simulink model "Senorless"  (R2023a)
settings: Solver=FixedStepDiscrete  StartTime=0.0  StopTime=5  FixedStep=1/FOC_FRQ  RelTol=1e-3
values from neighbouring files (symbols this model uses):
  ADC_REF = 3.6    [Senorless.sldd]
  ADC_SAMPLE_MAX = 32767.0    [Senorless.sldd]
  AMP_GAIN = 16.0    [Senorless.sldd]
  CURR_INPUT = 3276.0    [Senorless.sldd]
  CURR_KI = 380.0    [Senorless.sldd]
  CURR_KP = 0.04    [Senorless.sldd]
  CURR_LIMIT = 0.95    [Senorless.sldd]
  CURR_OVER = 6.0    [Senorless.sldd]
  CURR_POINT_GAIN = 7.0    [Senorless.sldd]
  CURR_STEP = 32760.0    [Senorless.sldd]
  CURR_UNDER = 0.03    [Senorless.sldd]
  CURR_WIDTH = 6552.0    [Senorless.sldd]
  FOC_FRQ = 25000.0    [Senorless.sldd]
  GAMMA = 32767.0    [Senorless.sldd]
  IMAX = 10.0    [Senorless.sldd]
  LPF_FRQ = 2000.0    [Senorless.sldd]
  MOTOR_DAMPER = 2.06E-7    [Senorless.sldd]
  MOTOR_FLUX = 0.00212352    [Senorless.sldd]
  MOTOR_INERTIA = 4.0E-7    [Senorless.sldd]
  MOTOR_LS = 0.000536    [Senorless.sldd]
  MOTOR_PN = 7.0    [Senorless.sldd]
  MOTOR_RS = 4.0    [Senorless.sldd]
  OPEN_IQ = 0.28    [Senorless.sldd]
  OPEN_IQ_MIN = 0.05    [Senorless.sldd]
  OPEN_IQ_SLOW = 0.1    [Senorless.sldd]
  OPEN_SPD = 1000.0    [Senorless.sldd]
  OPEN_SPD_SLOW = 180.0    [Senorless.sldd]
  OPEN_TIME = 0.5    [Senorless.sldd]
  OPEN_TIME_NFO = 0.5    [Senorless.sldd]
  PLL_LIMIT = 0.9    [Senorless.sldd]
  PLL_WIDTH = 800.0    [Senorless.sldd]
  PWM_FRQ = 96000000.0    [Senorless.sldd]
  RS_HUNT = 0.02    [Senorless.sldd]
  SMOK_FRQ = 600.0    [Senorless.sldd]
  SPD_LIMIT = 0.9    [Senorless.sldd]
  SPD_LPF_LEVEL = 0.0    [Senorless.sldd]
  SPD_MAX = 12000.0    [Senorless.sldd]
  SPD_MIN = 4000.0    [Senorless.sldd]
  SPD_REDUCE = 380.0    [Senorless.sldd]
  SPD_STEP = 6.0    [Senorless.sldd]
  SPD_WIDTH = 20.0    [Senorless.sldd]
  THETA_ERR_LIMIT = 8192.0    [Senorless.sldd]
  TS_POINT_GAIN = 10.0    [Senorless.sldd]
  UDC = 48.0    [Senorless.sldd]
  UDC_GAIN = 21.0    [Senorless.sldd]
  UDC_POINT_GAIN = 10.0    [Senorless.sldd]
undefined symbols (not defined in the file or in its folder): curr_q_ki, curr_q_kp, DiscIntNeverNeededParam, magnitude, PLL_LPF_LEVEL, Udc
libraries: simulink x20, slpidlib x5, mcbcontrolslib x2, mcbplantlib x1, autolibpmsmexterior x1, spspowerguiLib x1
(part 5 of 8)

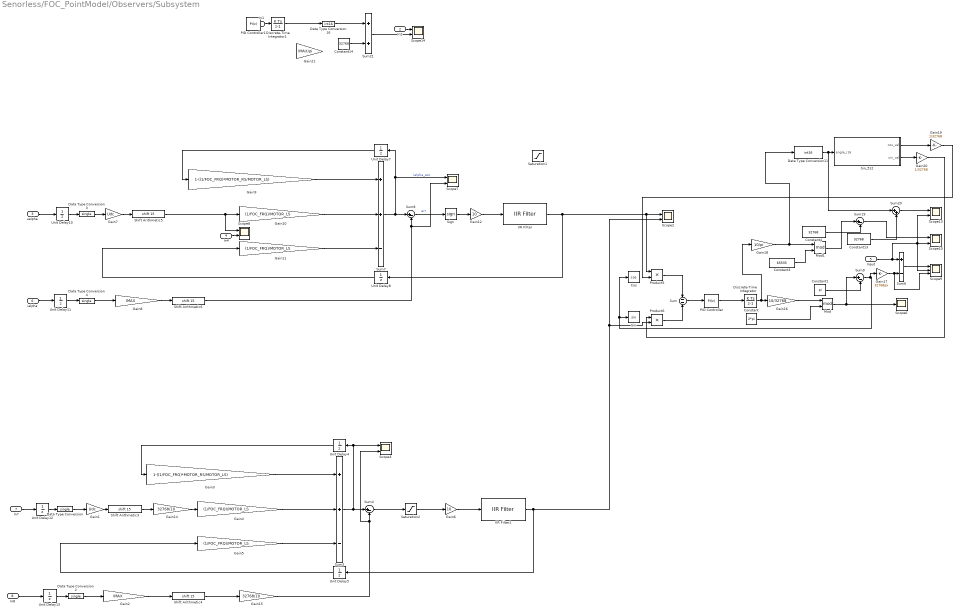
== system Senorless/FOC_PointModel/Observers/Subsystem ==
  In1 : Inport
  In2 : Inport  Port=2
  ualpha : Inport  Port=3
  In4 : Inport  Port=4
  Input : Inport  Port=5
  ialpha : Inport  Port=6
  In7 : Inport  Port=7
  In8 : Inport  Port=8
  Constant : Constant  Value=2*pi  OutDataTypeStr=single
  Constant1 : Constant  Value=pi  OutDataTypeStr=single
  Constant13 : Constant  Value=32768  OutDataTypeStr=int16
  Constant14 : Constant  Value=32768  OutDataTypeStr=int16
  Constant3 : Constant  Value=65535  OutDataTypeStr=single
  Constant4 : Constant  Value=32768
  Cos : Trigonometry  Operator=cos
  Data Type Conversion{,2..4} (4 alike) : DataTypeConversion  OutDataTypeStr=single  SaturateOnIntegerOverflow=off  RndMeth=Floor
  Data Type Conversion11 : DataTypeConversion  OutDataTypeStr=int16  SaturateOnIntegerOverflow=off  RndMeth=Floor
  Data Type Conversion16 : DataTypeConversion  OutDataTypeStr=int16  SaturateOnIntegerOverflow=off
  Discrete-Time Integrator : DiscreteIntegrator  SampleTime=-1  ICPrevOutput=DiscIntNeverNeededParam  ICPrevScaledInput=DiscIntNeverNeededParam
  Discrete-Time Integrator1 : DiscreteIntegrator  SampleTime=-1  OutDataTypeStr=int32  RndMeth=Zero  ICPrevOutput=DiscIntNeverNeededParam  ICPrevScaledInput=DiscIntNeverNeededParam
  Gain1 : Gain  Gain=Udc
  Gain10 : Gain  Gain=(1/FOC_FRQ)/MOTOR_LS
  Gain11 : Gain  Gain=(1/FOC_FRQ)/MOTOR_LS  OutDataTypeStr=single
  Gain12 : Gain  Gain=10
  Gain14 : Gain  Gain=32768/10
  Gain15 : Gain  Gain=32768/10
  Gain16 : Gain  Gain=10/32768
  Gain17 : Gain  Gain=32768/pi
  Gain18 : Gain  Gain=10/pi
  Gain19 : Gain  Gain=1/32768  OutDataTypeStr=single
  Gain2 : Gain  Gain=IMAX
  Gain20 : Gain  Gain=1/32768  OutDataTypeStr=single
  Gain21 : Gain  Gain=IMAX/pi  OutDataTypeStr=int32  RndMeth=Zero
  Gain3 : Gain  Gain=1-((1/FOC_FRQ)*MOTOR_RS/MOTOR_LS)  OutDataTypeStr=single
  Gain4 : Gain  Gain=(1/FOC_FRQ)/MOTOR_LS
  Gain5 : Gain  Gain=(1/FOC_FRQ)/MOTOR_LS  OutDataTypeStr=single
  Gain6 : Gain  Gain=10
  Gain7 : Gain  Gain=Udc
  Gain8 : Gain  Gain=IMAX
  Gain9 : Gain  Gain=1-((1/FOC_FRQ)*MOTOR_RS/MOTOR_LS)  OutDataTypeStr=single
  IIR Filter : mcbcontrolslib/IIR Filter  VariantControl=Low Pass Filter  VariantSelect=Low-pass  Filter_constant=0.1  advancedSettings=off  Ts=50e-6  cutOff_freq=353.6777
      settings: LibrarySourceBlock=mcbhdllib/Signal Management/IIR Filter
  IIR Filter1 : mcbcontrolslib/IIR Filter  VariantControl=Low Pass Filter  VariantSelect=Low-pass  Filter_constant=0.149  advancedSettings=off  Ts=50e-6  cutOff_freq=557.3228
      settings: LibrarySourceBlock=mcbhdllib/Signal Management/IIR Filter
  Mod : Math  Operator=mod
  Mod1 : Math  Operator=mod
  PID Controller : slpidlib/PID Controller  Controller=PI  Form=Parallel  TimeDomain=Discrete-time  UseExternalTs=off  SampleTime=-1  IntegratorMethod=Forward Euler  FilterMethod=Forward Euler  ControllerParametersSource=internal  P=2*0.707*100  I=100*100  UseKiTs=off  D=0  N=100  UseFilter=on  TunerSelectOption=Transfer Function Based (PID Tuner App)  InitialConditionSource=internal  InitialConditionForIntegrator=0  InitialConditionForFilter=0  DifferentiatorICPrevScaledInput=0  ExternalReset=none  TrackingMode=off  Kt=1  LimitOutput=off  SatLimitsSource=internal  UpperSaturationLimit=inf  LowerSaturationLimit=-inf  LinearizeAsGain=on  AntiWindupMode=none  Kb=1  LimitIntegrator=off  UpperIntegratorSaturationLimit=inf  LowerIntegratorSaturationLimit=-inf  POutMin=[]  POutMax=[]  IOutMin=[]  IOutMax=[]  DOutMin=[]  DOutMax=[]  NOutMin=[]  NOutMax=[]  SumOutMin=[]  SumOutMax=[]  SaturationOutMin=[]  SaturationOutMax=[]  PParamMin=[]  PParamMax=[]  IParamMin=[]  IParamMax=[]  DParamMin=[]  DParamMax=[]  NParamMin=[]  NParamMax=[]  KbParamMin=[]  KbParamMax=[]  KtParamMin=[]  KtParamMax=[]  KbOutMin=[]  KbOutMax=[]  KtOutMin=[]  KtOutMax=[]  IntegratorOutMin=[]  IntegratorOutMax=[]  FilterOutMin=[]  FilterOutMax=[]  SumI1OutMin=[]  SumI1OutMax=[]  SumI2OutMin=[]  SumI2OutMax=[]  SumI3OutMin=[]  SumI3OutMax=[]  SumI4OutMin=[]  SumI4OutMax=[]  SumDOutMin=[]  SumDOutMax=[]  DifferentiatorOutMin=[]  DifferentiatorOutMax=[]  FilterDiffOutCoefMin=[]  FilterDiffOutCoefMax=[]  ReciprocalOutMin=[]  ReciprocalOutMax=[]  SumDenOutMin=[]  SumDenOutMax=[]  SumNumOutMin=[]  SumNumOutMax=[]  DivideOutMin=[]  DivideOutMax=[]  UdiffTsProdOutMin=[]  UdiffTsProdOutMax=[]  NTsProdOutMin=[]  NTsProdOutMax=[]  UintegralTsProdOutMin=[]  UintegralTsProdOutMax=[]  UngainTsProdOutMin=[]  UngainTsProdOutMax=[]  ClampingZeroOutDataTypeStr=Inherit: Inherit via back propagation  ClampingZeroOutMin=[]  ClampingZeroOutMax=[]  FilterDenConstantOutDataTypeStr=Inherit: Inherit via back propagation  FilterDenConstantOutMin=[]  FilterDenConstantOutMax=[]  PCopyOutDataTypeStr=Inherit: Inherit via back propagation  PCopyOutMin=[]  PCopyOutMax=[]  NCopyOutDataTypeStr=Inherit: Inherit via back propagation  NCopyOutMin=[]  NCopyOutMax=[]  IntegratorContinuousStateAttributes=''  IntegratorStateMustResolveToSignalObject=off  IntegratorRTWStateStorageClass=Auto  FilterContinuousStateAttributes=''  FilterStateMustResolveToSignalObject=off  FilterRTWStateStorageClass=Auto  ParallelPVariant=InternalParameters  IdealPVariant=Disabled  IVariant=InternalParameters  DVariant=Disabled  IntegratorVariant=Discrete  SatVariant=Disabled  AWVariant=Passthrough  PCopyVariant=Disabled  TRVariant=Disabled  FdbkBlocksVariant=Forward  IdealPFdbkVariant=Disabled  SatFdbkVariant=Disabled  DerivativeFilterVariant=Disabled  NVariant=Disabled  NCopyVariant=Disabled_SignalSpec  FilterICVariant=Disabled  IntegratorICVariant=InternalICs  ExternalResetVariant=Disabled  TRSumVariant=Passthrough  SumFdbkVariant=Disabled  SumVariant=Sum_PI  TsampFilterVariant=InternalTs  TsampNgainVariant=Passthrough  TsampIntegralVariant=Disabled_SignalSpec  ExternalSaturationOutDataTypeStr=Inherit: Same as second input
  PID Controller1 : slpidlib/PID Controller  Controller=PI  Form=Parallel  TimeDomain=Discrete-time  UseExternalTs=off  SampleTime=-1  IntegratorMethod=Forward Euler  FilterMethod=Forward Euler  ControllerParametersSource=internal  P=2*0.707*100  I=100*100  UseKiTs=off  D=0  N=100  UseFilter=on  TunerSelectOption=Transfer Function Based (PID Tuner App)  InitialConditionSource=internal  InitialConditionForIntegrator=0  InitialConditionForFilter=0  DifferentiatorICPrevScaledInput=0  ExternalReset=none  TrackingMode=off  Kt=1  LimitOutput=off  SatLimitsSource=internal  UpperSaturationLimit=inf  LowerSaturationLimit=-inf  LinearizeAsGain=on  AntiWindupMode=none  Kb=1  LimitIntegrator=off  UpperIntegratorSaturationLimit=inf  LowerIntegratorSaturationLimit=-inf  PGainOutDataTypeStr=int32  PProdOutDataTypeStr=int32  POutMin=[]  POutMax=[]  IGainOutDataTypeStr=int32  IProdOutDataTypeStr=int32  IOutMin=[]  IOutMax=[]  DOutMin=[]  DOutMax=[]  NOutMin=[]  NOutMax=[]  SumOutDataTypeStr=int32  SumOutMin=[]  SumOutMax=[]  SaturationOutMin=[]  SaturationOutMax=[]  PParamDataTypeStr=int16  PParamMin=[]  PParamMax=[]  IParamDataTypeStr=int16  IParamMin=[]  IParamMax=[]  DParamMin=[]  DParamMax=[]  NParamMin=[]  NParamMax=[]  KbParamMin=[]  KbParamMax=[]  KtParamMin=[]  KtParamMax=[]  KbOutMin=[]  KbOutMax=[]  KtOutMin=[]  KtOutMax=[]  IntegratorOutDataTypeStr=int32  IntegratorOutMin=[]  IntegratorOutMax=[]  FilterOutMin=[]  FilterOutMax=[]  SumI1OutMin=[]  SumI1OutMax=[]  SumI2OutMin=[]  SumI2OutMax=[]  SumI3OutMin=[]  SumI3OutMax=[]  SumI4OutMin=[]  SumI4OutMax=[]  SumDOutMin=[]  SumDOutMax=[]  SumAccumDataTypeStr=int32  DifferentiatorOutMin=[]  DifferentiatorOutMax=[]  FilterDiffOutCoefMin=[]  FilterDiffOutCoefMax=[]  ReciprocalOutMin=[]  ReciprocalOutMax=[]  SumDenOutMin=[]  SumDenOutMax=[]  SumNumOutMin=[]  SumNumOutMax=[]  DivideOutMin=[]  DivideOutMax=[]  UdiffTsProdOutMin=[]  UdiffTsProdOutMax=[]  NTsProdOutMin=[]  NTsProdOutMax=[]  UintegralTsProdOutMin=[]  UintegralTsProdOutMax=[]  UngainTsProdOutMin=[]  UngainTsProdOutMax=[]  ClampingZeroOutDataTypeStr=Inherit: Inherit via back propagation  ClampingZeroOutMin=[]  ClampingZeroOutMax=[]  FilterDenConstantOutDataTypeStr=Inherit: Inherit via back propagation  FilterDenConstantOutMin=[]  FilterDenConstantOutMax=[]  PCopyOutDataTypeStr=Inherit: Inherit via back propagation  PCopyOutMin=[]  PCopyOutMax=[]  NCopyOutDataTypeStr=Inherit: Inherit via back propagation  NCopyOutMin=[]  NCopyOutMax=[]  IntegratorContinuousStateAttributes=''  IntegratorStateMustResolveToSignalObject=off  IntegratorRTWStateStorageClass=Auto  FilterContinuousStateAttributes=''  FilterStateMustResolveToSignalObject=off  FilterRTWStateStorageClass=Auto  ParallelPVariant=InternalParameters  IdealPVariant=Disabled  IVariant=InternalParameters  DVariant=Disabled  IntegratorVariant=Discrete  SatVariant=Disabled  AWVariant=Passthrough  PCopyVariant=Disabled  TRVariant=Disabled  FdbkBlocksVariant=Forward  IdealPFdbkVariant=Disabled  SatFdbkVariant=Disabled  DerivativeFilterVariant=Disabled  NVariant=Disabled  NCopyVariant=Disabled_SignalSpec  FilterICVariant=Disabled  IntegratorICVariant=InternalICs  ExternalResetVariant=Disabled  TRSumVariant=Passthrough  SumFdbkVariant=Disabled  SumVariant=Sum_PI  TsampFilterVariant=InternalTs  TsampNgainVariant=Passthrough  TsampIntegralVariant=Disabled_SignalSpec  ExternalSaturationOutDataTypeStr=Inherit: Same as second input
  Product5 : Product
  Product6 : Product
  Saturation1 : Saturate  UpperLimit=32768  LowerLimit=-32768
  Saturation2 : Saturate  UpperLimit=32768  LowerLimit=-32768
  Scope{2..3,7..8,10,13..14} (7 alike) : Scope  NumInputPorts=2
  Scope6 : Scope
  Scope9 : Scope  NumInputPorts=3
  Shift Arithmetic{3..6} (4 alike) : ArithShift  BitShiftNumber=15
  Sign : Signum
  Sin : Trigonometry
  Sin_512 : MATLAB Function  TreatAsAtomicUnit=on
  Sum : Sum  Inputs=--
  Sum19 : Sum  Inputs=|+-
  Sum20 : Sum  Inputs=|++
  Sum21 : Sum
  Sum3 : Sum  Inputs=++-
  Sum4 : Sum  Inputs=|+-  RndMeth=Zero
  Sum6 : Sum  Inputs=+-
  Sum7 : Sum  Inputs=++-
  Sum8 : Sum  Inputs=|+-  RndMeth=Zero
  Sum9 : Sum  Inputs=|+-
  Unit Delay{4..5,7..8,10..13} (8 alike) : UnitDelay  SampleTime=-1  HasFrameUpgradeWarning=on
  wires:
  Sum8/1 -> Sign/1  "err"
  Gain3/1 -> Sum3/1
  Sum9/1 -> Cos/1, Sin/1, Gain17/1
  Saturation2/1 -> Gain6/1
  Unit Delay11/1 -> Data Type Conversion4/1
  Sum7/1 -> Unit Delay7/1, Scope7/1, Sum8/1  "ialpha_est"
  IIR Filter1/1 -> Unit Delay5/1, Scope2/2, Product6/2
  Data Type Conversion4/1 -> Gain8/1
  Unit Delay10/1 -> Data Type Conversion3/1
  Gain18/1 -> Mod1/1, Data Type Conversion11/1
  Gain20/1 -> Product6/1
  Sin_512/1(cos_val) -> Gain19/1
  Product5/1 -> Sum/1
  Gain15/1 -> Scope3/2, Sum4/2
  Sum4/1 -> Saturation2/1
  Input/1 -> Scope13/2, Scope9/2, Scope10/2, Sum6/1
  Gain4/1 -> Sum3/2
  Shift Arithmetic3/1 -> Gain14/1
  Gain2/1 -> Shift Arithmetic4/1
  Shift Arithmetic5/1 -> Scope8/1, Gain10/1
  Sum3/1 -> Scope3/1, Unit Delay4/1, Sum4/1
  Data Type Conversion3/1 -> Gain7/1
  Constant14/1 -> Sum21/2
  Unit Delay4/1 -> Gain3/1
  Gain1/1 -> Shift Arithmetic3/1
  Gain10/1 -> Sum7/2
  Discrete-Time Integrator1/1 -> Data Type Conversion16/1
  Sum21/1 -> Scope14/2
  Shift Arithmetic6/1 -> Scope7/2, Sum8/2
  Data Type Conversion/1 -> Gain1/1
  Shift Arithmetic4/1 -> Gain15/1
  Sign/1 -> Gain12/1
  Constant3/1 -> Mod1/2
  Gain8/1 -> Shift Arithmetic6/1
  Gain11/1 -> Sum7/3
  Unit Delay12/1 -> Data Type Conversion/1
  ialpha/1 -> Unit Delay11/1
  Unit Delay7/1 -> Gain9/1
  Unit Delay13/1 -> Data Type Conversion2/1
  Data Type Conversion2/1 -> Gain2/1
  Sum19/1 -> Scope10/1
  Gain5/1 -> Sum3/3
  Gain7/1 -> Shift Arithmetic5/1
  Constant/1 -> Mod/2
  Unit Delay5/1 -> Gain5/1
  ualpha/1 -> Unit Delay10/1
  Unit Delay8/1 -> Gain11/1
  Gain9/1 -> Sum7/1
  Mod/1 -> Sum9/1, Scope6/1
  Discrete-Time Integrator/1 -> Gain18/1, Gain16/1
  Gain17/1 -> Scope9/3, Sum6/2
  Constant4/1 -> Sum19/2
  IIR Filter/1 -> Unit Delay8/1, Product5/1, Scope2/1
  PID Controller/1 -> Discrete-Time Integrator/1
  Gain16/1 -> Mod/1
  Data Type Conversion16/1 -> Sum21/1
  Sin_512/2(sin_val) -> Gain20/1
  Constant1/1 -> Sum9/2
  Mod1/1 -> Sum19/1
  Gain19/1 -> Product5/2
  Constant13/1 -> Sum20/2
  Sum6/1 -> Scope9/1
  Gain6/1 -> IIR Filter1/1
  Data Type Conversion11/1 -> Sum20/1, Sin_512/1(angle_i16)
  Gain12/1 -> IIR Filter/1
  Sum20/1 -> Scope13/1
  Gain14/1 -> Gain4/1
  In2/1 -> Scope14/1
  Product6/1 -> Sum/2
  Sum/1 -> PID Controller/1
  In4/1 -> Scope8/2
  In7/1 -> Unit Delay12/1
  In8/1 -> Unit Delay13/1
  In1/1 -> Discrete-Time Integrator1/1

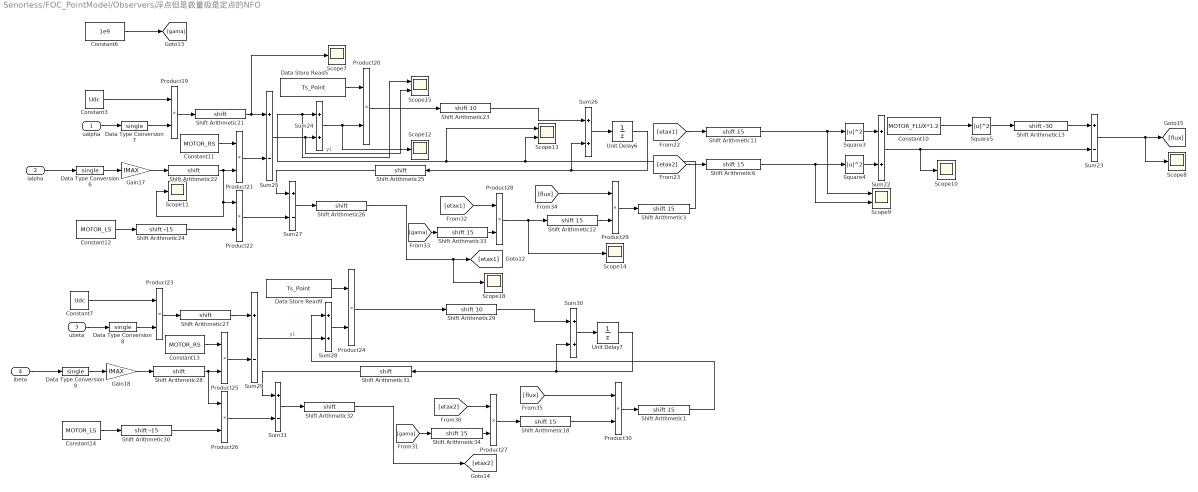
== system Senorless/FOC_PointModel/Observers/浮点但是数量级是定点的NFO ==
  ualpha : Inport
  ialpha : Inport  Port=2
  ubeta : Inport  Port=3
  ibeta : Inport  Port=4
  Constant10 : Constant  Value=MOTOR_FLUX*1.2  OutDataTypeStr=single
  Constant11 : Constant  Value=MOTOR_RS  OutDataTypeStr=single
  Constant12 : Constant  Value=MOTOR_LS  OutDataTypeStr=single
  Constant13 : Constant  Value=MOTOR_RS  OutDataTypeStr=single
  Constant14 : Constant  Value=MOTOR_LS  OutDataTypeStr=single
  Constant3 : Constant  Value=Udc  OutDataTypeStr=single
  Constant6 : Constant  Value=1e9  OutDataTypeStr=uint32
  Constant7 : Constant  Value=Udc  OutDataTypeStr=single
  Data Store Read5 : DataStoreRead  DataStoreName=Ts_Point  IndexOptions=Index vector (dialog)  Indices=1  OutputSizes=1
  Data Store Read9 : DataStoreRead  DataStoreName=Ts_Point  IndexOptions=Index vector (dialog)  Indices=1  OutputSizes=1
  Data Type Conversion{6..9} (4 alike) : DataTypeConversion  OutDataTypeStr=single  SaturateOnIntegerOverflow=off  RndMeth=Floor
  Gain17 : Gain  Gain=IMAX  ParamDataTypeStr=single  OutDataTypeStr=single  RndMeth=Zero
  Gain18 : Gain  Gain=IMAX  ParamDataTypeStr=int16  OutDataTypeStr=single  RndMeth=Zero
  Product{19..30} (12 alike) : Product  OutDataTypeStr=single  RndMeth=Zero
  Scope{7..8,10..12,14,18} (7 alike) : Scope
  Scope13 : Scope  NumInputPorts=2
  Scope15 : Scope  NumInputPorts=2
  Scope9 : Scope  NumInputPorts=2
  Shift Arithmetic{1,3,6,11..12,18,33..34} (8 alike) : ArithShift  BitShiftNumber=15
  Shift Arithmetic13 : ArithShift  BitShiftNumber=-30
  Shift Arithmetic{21..22,25..28,31..32} (8 alike) : ArithShift
  Shift Arithmetic23 : ArithShift  BitShiftNumber=10
  Shift Arithmetic24 : ArithShift  BitShiftNumber=-15
  Shift Arithmetic29 : ArithShift  BitShiftNumber=10
  Shift Arithmetic30 : ArithShift  BitShiftNumber=-15
  Square3 : Math  Operator=magnitude^2
  Square4 : Math  Operator=magnitude^2
  Square5 : Math  Operator=magnitude^2
  Sum{22,24,26,28,30} (5 alike) : Sum  OutDataTypeStr=single  RndMeth=Zero
  Sum{23,25,27,29,31} (5 alike) : Sum  Inputs=+-  OutDataTypeStr=single  RndMeth=Zero
  Unit Delay6 : UnitDelay  SampleTime=-1  HasFrameUpgradeWarning=on
  Unit Delay7 : UnitDelay  SampleTime=-1  HasFrameUpgradeWarning=on
  wires:
  Product25/1 -> Sum29/2
  Shift Arithmetic29/1 -> Sum30/1
  Product24/1 -> Shift Arithmetic29/1
  Product26/1 -> Sum31/2
  Unit Delay6/1 -> Sum26/2, Shift Arithmetic25/1
  Gain17/1 -> Shift Arithmetic22/1
  Shift Arithmetic11/1 -> Scope9/1, Square3/1
  Constant7/1 -> Product23/1
  Shift Arithmetic13/1 -> Sum23/1
  Gain18/1 -> Shift Arithmetic28/1
  Sum31/1 -> Shift Arithmetic32/1
  Shift Arithmetic3/1 -> Scope13/1, Scope15/1, Sum24/1, Scope13/2
  Shift Arithmetic28/1 -> Product26/1, Product25/2
  Unit Delay7/1 -> Sum30/2, Shift Arithmetic31/1
  Sum22/1 -> Scope10/1, Sum23/2
  Sum29/1 -> Sum28/2  "y1"
  Data Type Conversion6/1 -> Gain17/1
  Shift Arithmetic27/1 -> Sum29/1
  [flux] -> Product30/1
  Data Type Conversion8/1 -> Product23/2
  Shift Arithmetic23/1 -> Sum26/1
  Constant13/1 -> Product25/1
  Sum23/1 -> Scope8/1, [flux]
  Product27/1 -> Shift Arithmetic18/1
  Data Store Read9/1 -> Product24/1
  Sum28/1 -> Product24/2
  Sum24/1 -> Scope12/1, Product20/2
  Constant14/1 -> Shift Arithmetic30/1
  Sum30/1 -> Unit Delay7/1
  Shift Arithmetic25/1 -> Sum27/1
  Constant12/1 -> Shift Arithmetic24/1
  Shift Arithmetic31/1 -> Sum31/1
  Constant3/1 -> Product19/1
  Product23/1 -> Shift Arithmetic27/1
  Shift Arithmetic6/1 -> Scope9/2, Square4/1
  Shift Arithmetic34/1 -> Product27/2
  Square5/1 -> Shift Arithmetic13/1
  Square3/1 -> Sum22/1
  Product19/1 -> Shift Arithmetic21/1
  Sum26/1 -> Unit Delay6/1
  [etax1] -> Product28/1
  Sum27/1 -> Shift Arithmetic26/1
  Product29/1 -> Shift Arithmetic3/1
  Shift Arithmetic12/1 -> Product29/2
  ibeta/1 -> Data Type Conversion9/1
  [flux] -> Product29/1
  Constant11/1 -> Product21/1
  Product28/1 -> Scope14/1, Shift Arithmetic12/1
  Product22/1 -> Sum27/2
  Shift Arithmetic32/1 -> [etax2]
  Product21/1 -> Sum25/2
  Shift Arithmetic22/1 -> Product22/1, Scope11/1, Product21/2
  Shift Arithmetic33/1 -> Product28/2
  Sum25/1 -> Scope15/2, Sum24/2  "y1"
  [gama] -> Shift Arithmetic34/1
  Square4/1 -> Sum22/2
  Product20/1 -> Shift Arithmetic23/1
  ualpha/1 -> Data Type Conversion7/1
  [gama] -> Shift Arithmetic33/1
  Constant10/1 -> Square5/1
  Shift Arithmetic18/1 -> Product30/2
  Shift Arithmetic26/1 -> Scope18/1, [etax1]
  [etax2] -> Product27/1
  [etax1] -> Shift Arithmetic11/1
  Data Type Conversion9/1 -> Gain18/1
  ialpha/1 -> Data Type Conversion6/1
  Shift Arithmetic21/1 -> Scope7/1, Sum25/1
  Shift Arithmetic30/1 -> Product26/2
  Product30/1 -> Shift Arithmetic1/1
  Shift Arithmetic24/1 -> Product22/2
  [etax2] -> Shift Arithmetic6/1
  Shift Arithmetic1/1 -> Sum28/1
  Data Type Conversion7/1 -> Product19/2
  ubeta/1 -> Data Type Conversion8/1
  Data Store Read5/1 -> Product20/1
  Constant6/1 -> [gama]

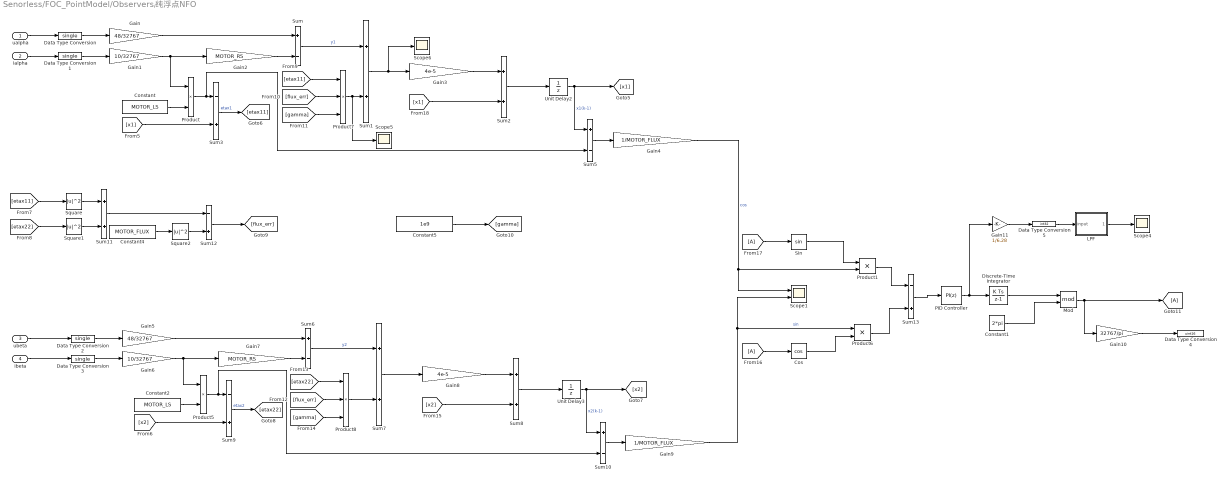
== system Senorless/FOC_PointModel/Observers/纯浮点NFO ==
  ualpha : Inport
  ialpha : Inport  Port=2
  ubeta : Inport  Port=3
  ibeta : Inport  Port=4
  Constant : Constant  Value=MOTOR_LS
  Constant1 : Constant  Value=2*pi  OutDataTypeStr=single
  Constant2 : Constant  Value=MOTOR_LS
  Constant4 : Constant  Value=MOTOR_FLUX
  Constant5 : Constant  Value=1e9  OutDataTypeStr=single
  Cos : Trigonometry  Operator=cos
  Data Type Conversion{,1..3} (4 alike) : DataTypeConversion  OutDataTypeStr=single  SaturateOnIntegerOverflow=off  RndMeth=Floor
  Data Type Conversion4 : DataTypeConversion  OutDataTypeStr=uint16  SaturateOnIntegerOverflow=off  RndMeth=Floor
  Data Type Conversion5 : DataTypeConversion  OutDataTypeStr=int32  SaturateOnIntegerOverflow=off  RndMeth=Floor
  Discrete-Time Integrator : DiscreteIntegrator  SampleTime=-1  ICPrevOutput=DiscIntNeverNeededParam  ICPrevScaledInput=DiscIntNeverNeededParam
  From16 : From
  From17 : From
  Gain : Gain  Gain=48/32767
  Gain1 : Gain  Gain=10/32767
  Gain10 : Gain  Gain=32767/pi
  Gain11 : Gain  Gain=1/6.28
  Gain2 : Gain  Gain=MOTOR_RS
  Gain3 : Gain  Gain=4e-5  OutDataTypeStr=single
  Gain4 : Gain  Gain=1/MOTOR_FLUX
  Gain5 : Gain  Gain=48/32767
  Gain6 : Gain  Gain=10/32767
  Gain7 : Gain  Gain=MOTOR_RS
  Gain8 : Gain  Gain=4e-5  OutDataTypeStr=single
  Gain9 : Gain  Gain=1/MOTOR_FLUX
  Goto11 : Goto
  LPF : Subsystem  TreatAsAtomicUnit=on
  Mod : Math  Operator=mod
  PID Controller : slpidlib/PID Controller  Controller=PI  Form=Parallel  TimeDomain=Discrete-time  UseExternalTs=off  SampleTime=-1  IntegratorMethod=Forward Euler  FilterMethod=Forward Euler  ControllerParametersSource=internal  P=2*800  I=800*800  UseKiTs=off  D=0  N=100  UseFilter=on  TunerSelectOption=Transfer Function Based (PID Tuner App)  InitialConditionSource=internal  InitialConditionForIntegrator=0  InitialConditionForFilter=0  DifferentiatorICPrevScaledInput=0  ExternalReset=none  TrackingMode=off  Kt=1  LimitOutput=off  SatLimitsSource=internal  UpperSaturationLimit=inf  LowerSaturationLimit=-inf  LinearizeAsGain=on  AntiWindupMode=none  Kb=1  LimitIntegrator=off  UpperIntegratorSaturationLimit=inf  LowerIntegratorSaturationLimit=-inf  POutMin=[]  POutMax=[]  IOutMin=[]  IOutMax=[]  DOutMin=[]  DOutMax=[]  NOutMin=[]  NOutMax=[]  SumOutMin=[]  SumOutMax=[]  SaturationOutMin=[]  SaturationOutMax=[]  PParamMin=[]  PParamMax=[]  IParamMin=[]  IParamMax=[]  DParamMin=[]  DParamMax=[]  NParamMin=[]  NParamMax=[]  KbParamMin=[]  KbParamMax=[]  KtParamMin=[]  KtParamMax=[]  KbOutMin=[]  KbOutMax=[]  KtOutMin=[]  KtOutMax=[]  IntegratorOutMin=[]  IntegratorOutMax=[]  FilterOutMin=[]  FilterOutMax=[]  SumI1OutMin=[]  SumI1OutMax=[]  SumI2OutMin=[]  SumI2OutMax=[]  SumI3OutMin=[]  SumI3OutMax=[]  SumI4OutMin=[]  SumI4OutMax=[]  SumDOutMin=[]  SumDOutMax=[]  DifferentiatorOutMin=[]  DifferentiatorOutMax=[]  FilterDiffOutCoefMin=[]  FilterDiffOutCoefMax=[]  ReciprocalOutMin=[]  ReciprocalOutMax=[]  SumDenOutMin=[]  SumDenOutMax=[]  SumNumOutMin=[]  SumNumOutMax=[]  DivideOutMin=[]  DivideOutMax=[]  UdiffTsProdOutMin=[]  UdiffTsProdOutMax=[]  NTsProdOutMin=[]  NTsProdOutMax=[]  UintegralTsProdOutMin=[]  UintegralTsProdOutMax=[]  UngainTsProdOutMin=[]  UngainTsProdOutMax=[]  ClampingZeroOutDataTypeStr=Inherit: Inherit via back propagation  ClampingZeroOutMin=[]  ClampingZeroOutMax=[]  FilterDenConstantOutDataTypeStr=Inherit: Inherit via back propagation  FilterDenConstantOutMin=[]  FilterDenConstantOutMax=[]  PCopyOutDataTypeStr=Inherit: Inherit via back propagation  PCopyOutMin=[]  PCopyOutMax=[]  NCopyOutDataTypeStr=Inherit: Inherit via back propagation  NCopyOutMin=[]  NCopyOutMax=[]  IntegratorContinuousStateAttributes=''  IntegratorStateMustResolveToSignalObject=off  IntegratorRTWStateStorageClass=Auto  FilterContinuousStateAttributes=''  FilterStateMustResolveToSignalObject=off  FilterRTWStateStorageClass=Auto  ParallelPVariant=InternalParameters  IdealPVariant=Disabled  IVariant=InternalParameters  DVariant=Disabled  IntegratorVariant=Discrete  SatVariant=Disabled  AWVariant=Passthrough  PCopyVariant=Disabled  TRVariant=Disabled  FdbkBlocksVariant=Forward  IdealPFdbkVariant=Disabled  SatFdbkVariant=Disabled  DerivativeFilterVariant=Disabled  NVariant=Disabled  NCopyVariant=Disabled_SignalSpec  FilterICVariant=Disabled  IntegratorICVariant=InternalICs  ExternalResetVariant=Disabled  TRSumVariant=Passthrough  SumFdbkVariant=Disabled  SumVariant=Sum_PI  TsampFilterVariant=InternalTs  TsampNgainVariant=Passthrough  TsampIntegralVariant=Disabled_SignalSpec  ExternalSaturationOutDataTypeStr=Inherit: Same as second input
  Product{,1,5..6} (4 alike) : Product
  Product7 : Product  Inputs=3
  Product8 : Product  Inputs=3
  Scope1 : Scope  NumInputPorts=2
  Scope4 : Scope
  Scope5 : Scope
  Scope6 : Scope
  Sin : Trigonometry
  Square : Math  Operator=magnitude^2  OutputSignalType=real
  Square1 : Math  Operator=magnitude^2  OutputSignalType=real
  Square2 : Math  Operator=magnitude^2  OutputSignalType=real
  Sum{,5..6,10} (4 alike) : Sum  Inputs=+-
  Sum{1..2,7..8,11} (5 alike) : Sum
  Sum{3,9,12..13} (4 alike) : Sum  Inputs=-+
  Unit Delay2 : UnitDelay  SampleTime=-1  HasFrameUpgradeWarning=on
  Unit Delay3 : UnitDelay  SampleTime=-1  HasFrameUpgradeWarning=on
  wires:
  Gain8/1 -> Sum8/1
  Constant2/1 -> Product5/2
  Sum/1 -> Sum1/1  "y1"
  Sum2/1 -> Unit Delay2/1
  Sum10/1 -> Gain9/1
  Gain4/1 -> Scope1/1, Product1/2  "cos"
  [x1] -> Sum2/2
  ibeta/1 -> Data Type Conversion3/1
  ubeta/1 -> Data Type Conversion2/1
  [etax22] -> Square1/1
  Data Type Conversion/1 -> Gain/1
  [etax11] -> Square/1
  Sum9/1 -> [etax22]  "etax2"
  Gain/1 -> Sum/1
  Product5/1 -> Sum10/2, Sum9/1
  Square2/1 -> Sum12/2
  Product1/1 -> Sum13/1
  Gain5/1 -> Sum6/1
  Sum1/1 -> Scope6/1, Gain3/1
  Data Type Conversion3/1 -> Gain6/1
  Sum8/1 -> Unit Delay3/1
  [flux_err] -> Product8/2
  Sum5/1 -> Gain4/1
  PID Controller/1 -> Gain11/1, Discrete-Time Integrator/1
  Cos/1 -> Product6/2
  [etax22] -> Product8/1
  [gamma] -> Product7/3
  Square1/1 -> Sum11/2
  [x1] -> Sum3/2
  Constant/1 -> Product/2
  Product7/1 -> Scope5/1, Sum1/2
  Sum13/1 -> PID Controller/1
  Square/1 -> Sum11/1
  Sum6/1 -> Sum7/1  "y2"
  Product8/1 -> Sum7/2
  Discrete-Time Integrator/1 -> Mod/1
  [flux_err] -> Product7/2
  Constant5/1 -> [gamma]
  Constant4/1 -> Square2/1
  Sum12/1 -> [flux_err]
  [gamma] -> Product8/3
  Sum3/1 -> [etax11]  "etax1"
  Gain9/1 -> Scope1/2, Product6/1  "sin"
  [etax11] -> Product7/1
  Gain7/1 -> Sum6/2
  Gain1/1 -> Product/1, Gain2/1
  Gain10/1 -> Data Type Conversion4/1
  ialpha/1 -> Data Type Conversion1/1
  Gain6/1 -> Gain7/1, Product5/1
  Gain3/1 -> Sum2/1
  Sin/1 -> Product1/1
  Product6/1 -> Sum13/2
  Sum11/1 -> Sum12/1
  From17/1 -> Sin/1
  Data Type Conversion1/1 -> Gain1/1
  Gain11/1 -> Data Type Conversion5/1
  Mod/1 -> Gain10/1, Goto11/1
  From16/1 -> Cos/1
  Constant1/1 -> Mod/2
  [x2] -> Sum8/2
  Gain2/1 -> Sum/2
  [x2] -> Sum9/2
  Data Type Conversion2/1 -> Gain5/1
  Sum7/1 -> Gain8/1
  Unit Delay3/1 -> Sum10/1, [x2]  "x2(k-1)"
  Unit Delay2/1 -> Sum5/1, [x1]  "x1(k-1)"
  Product/1 -> Sum5/2, Sum3/1
  LPF/1(output) -> Scope4/1
  Data Type Conversion5/1 -> LPF/1(input)
  ualpha/1 -> Data Type Conversion/1

== system Senorless/FOC_PointModel/SVPWM/AntiClark ==
  note: Va = Valpha;
      | Vb = Valpha*(-1/2)+Vbeta*sqrt(3)/2
      | Vc = Valpha*(-1/2)-Vbeta*sqrt(3)/2
  Valpha : Inport
  Vbeta : Inport  Port=2
  Gain1 : Gain  Gain=32767*sqrt(3)/2  ParamDataTypeStr=int16  OutDataTypeStr=int32  RndMeth=Zero
  Shift Arithmetic : ArithShift  BitShiftNumber=15
  Shift Arithmetic1 : ArithShift  BitShiftNumber=1
  Sum : Sum  Inputs=|-+  RndMeth=Zero
  Sum1 : Sum  Inputs=--|  RndMeth=Zero
  Va : Outport
  Vb : Outport  Port=2
  Vc : Outport  Port=3
  wires:
  Vbeta/1 -> Gain1/1
  Shift Arithmetic1/1 -> Sum1/2, Sum/1
  Sum/1 -> Vb/1
  Gain1/1 -> Shift Arithmetic/1
  Sum1/1 -> Vc/1
  Shift Arithmetic/1 -> Sum1/1, Sum/2
  Valpha/1 -> Va/1, Shift Arithmetic1/1

== system Senorless/FOC_PointModel/SVPWM/ei_t ==
  note: V0 = -1/2(Vmax+Vmin)
  Vabc : Inport
  Demux : Demux  Outputs=3
  Min : MinMax  Inputs=3  RndMeth=Zero
  Min1 : MinMax  Function=max  Inputs=3  RndMeth=Zero
  Shift Arithmetic : ArithShift  BitShiftNumber=1
  Sum : Sum  Inputs=|++  OutDataTypeStr=int32  RndMeth=Zero
  Unary Minus : UnaryMinus
  ei_t : Outport
  wires:
  Min/1 -> Sum/1
  Sum/1 -> Shift Arithmetic/1
  Min1/1 -> Sum/2
  Shift Arithmetic/1 -> Unary Minus/1
  Vabc/1 -> Demux/1
  Demux/1 -> Min1/1, Min/1
  Demux/2 -> Min/2, Min1/2
  Demux/3 -> Min1/3, Min/3
  Unary Minus/1 -> ei_t/1

== system Senorless/FOC_PointModel/idq_Controller/PI Controller ==
  input : Inport
  Kp : Inport  Port=2
  Ki : Inport  Port=3
  Data Store Read3 : DataStoreRead  DataStoreName=Curr_Limit  IndexOptions=Index vector (dialog)  Indices=1  OutputSizes=1
  Gain : Gain  Gain=-1  OutDataTypeStr=int32  RndMeth=Zero
  Product2 : Product  OutDataTypeStr=int32  RndMeth=Zero
  Saturation Dynamic2 : simulink/Discontinuities/Saturation Dynamic  OutMin=[]  OutMax=[]  OutDataTypeStr=Inherit: Same as second input  OutDataType=fixdt(1, 16)  OutScaling=2^-10  RndMeth=Zero  DoSatur=off
  Scope : Scope  NumInputPorts=2
  Sum : Sum  OutDataTypeStr=int32  RndMeth=Zero
  input1 : InportShadow
  积分器 : Subsystem
      settings: MinAlgLoopOccurrences=on
  output : Outport
  wires:
  input/1 -> Product2/1
  Kp/1 -> Product2/2
  Ki/1 -> 积分器/1(Ki)
  input1/1 -> 积分器/2(input)
  Product2/1 -> Scope/1, Sum/1
  积分器/1(output) -> Sum/2, Scope/2
  Sum/1 -> Saturation Dynamic2/2
  Saturation Dynamic2/1 -> output/1
  Data Store Read3/1 -> [limit]
  [limit] -> Gain/1
  Gain/1 -> Saturation Dynamic2/3
  [limit] -> Saturation Dynamic2/1

== system Senorless/FOC_PointModel/idq_Controller/PI Controller1 ==
  Ki : Inport
  Kp : Inport  Port=2
  input : Inport  Port=3
  Data Store Read3 : DataStoreRead  DataStoreName=Curr_Limit  IndexOptions=Index vector (dialog)  Indices=1  OutputSizes=1
  Gain : Gain  Gain=-1  OutDataTypeStr=int32  RndMeth=Zero
  Product2 : Product  OutDataTypeStr=int32  RndMeth=Zero
  Saturation Dynamic2 : simulink/Discontinuities/Saturation Dynamic  OutMin=[]  OutMax=[]  OutDataTypeStr=Inherit: Same as second input  OutDataType=fixdt(1, 16)  OutScaling=2^-10  RndMeth=Zero  DoSatur=off
  Scope : Scope  NumInputPorts=2
  Sum : Sum  OutDataTypeStr=int32  RndMeth=Zero
  input1 : InportShadow  Port=3
  积分器 : Subsystem
      settings: MinAlgLoopOccurrences=on
  output : Outport
  wires:
  [limit] -> Saturation Dynamic2/1
  Gain/1 -> Saturation Dynamic2/3
  [limit] -> Gain/1
  Data Store Read3/1 -> [limit]
  Saturation Dynamic2/1 -> output/1
  Sum/1 -> Saturation Dynamic2/2
  积分器/1(output) -> Scope/2, Sum/2
  Product2/1 -> Sum/1, Scope/1
  input1/1 -> 积分器/2(input)
  Ki/1 -> 积分器/1(Ki)
  Kp/1 -> Product2/2
  input/1 -> Product2/1

== system Senorless/FOC_PointModel/idq_Controller/PI Controller2 ==
  input : Inport
  Kp : Inport  Port=2
  Ki : Inport  Port=3
  Reset : Inport  Port=4
  Xo : Inport  Port=5
  Action Port : ActionPort  InitializeStates=reset  ActionPortLabel=if(u1 > 0)
  Data Store Read3 : DataStoreRead  DataStoreName=Curr_Limit  IndexOptions=Index vector (dialog)  Indices=1  OutputSizes=1
  Gain : Gain  Gain=-1  OutDataTypeStr=int32  RndMeth=Zero
  MATLAB Function : MATLAB Function  TreatAsAtomicUnit=on
  Product2 : Product  OutDataTypeStr=int32  RndMeth=Zero
  Scope : Scope  NumInputPorts=2
  Sum : Sum  OutDataTypeStr=int32  RndMeth=Zero
  input1 : InportShadow
  积分器/双边沿初始化 : Subsystem
      settings: MinAlgLoopOccurrences=on
  output : Outport
  wires:
  [limit] -> MATLAB Function/2(up), Gain/1
  Gain/1 -> MATLAB Function/3(low)
  Data Store Read3/1 -> [limit]
  MATLAB Function/1(out) -> output/1
  Sum/1 -> MATLAB Function/1(in)
  积分器/双边沿初始化/1(output) -> Scope/2, Sum/2
  Product2/1 -> Sum/1, Scope/1
  input1/1 -> 积分器/双边沿初始化/2(input)
  Reset/1 -> 积分器/双边沿初始化/4(Reset)
  Xo/1 -> 积分器/双边沿初始化/3(Xo)
  Ki/1 -> 积分器/双边沿初始化/1(Ki)
  Kp/1 -> Product2/2
  input/1 -> Product2/1

== system Senorless/FOC_PointModel/加速强拖/FreqGenerator_point2 ==
  Freq : Inport
  Reset : Inport  Port=2
  Constant : Constant  Value=32768  OutDataTypeStr=int16
  Data Type Conversion : DataTypeConversion  OutDataTypeStr=int16  SaturateOnIntegerOverflow=off
  Data Type Conversion1 : DataTypeConversion  OutDataTypeStr=int16  SaturateOnIntegerOverflow=off
  Discrete-Time Integrator : DiscreteIntegrator  ExternalReset=rising  SampleTime=-1  OutDataTypeStr=int32  RndMeth=Zero  ICPrevOutput=DiscIntNeverNeededParam  ICPrevScaledInput=DiscIntNeverNeededParam
  Discrete-Time Integrator1 : DiscreteIntegrator  ExternalReset=rising  SampleTime=-1  OutDataTypeStr=int32  RndMeth=Zero  ICPrevOutput=DiscIntNeverNeededParam  ICPrevScaledInput=DiscIntNeverNeededParam
  Gain6 : Gain  Gain=65535  OutDataTypeStr=int32  RndMeth=Zero
  Scope : Scope
  Scope1 : Scope
  Scope2 : Scope
  Shift Arithmetic : ArithShift  BitShiftNumber=-8
  Shift Arithmetic1 : ArithShift  BitShiftNumber=8
  Theta : Outport
  wires:
  Freq/1 -> Data Type Conversion1/1
  Gain6/1 -> Shift Arithmetic/1
  Data Type Conversion1/1 -> Gain6/1
  Discrete-Time Integrator/1 -> Scope2/1, Scope/1, Shift Arithmetic1/1
  Shift Arithmetic1/1 -> Data Type Conversion/1
  Reset/1 -> Discrete-Time Integrator1/2, Discrete-Time Integrator/2
  Discrete-Time Integrator1/1 -> Scope1/1, Discrete-Time Integrator/1
  Shift Arithmetic/1 -> Discrete-Time Integrator1/1
  Data Type Conversion/1 -> Theta/1

== system Senorless/FOC_PointModel/加速强拖/Subsystem ==
  Open_Hz : Inport
  Reset : Inport  Port=2
  Constant1 : Constant  Value=0  OutDataTypeStr=int32
  Gain : Gain  Gain=256  OutDataTypeStr=int32  RndMeth=Zero
  Saturation : Saturate  UpperLimit=1  LowerLimit=-1
  Sum : Sum  Inputs=-+|
  Sum1 : Sum  Inputs=++|  RndMeth=Zero
  Switch : Switch  Threshold=1  OutDataTypeStr=int32  RndMeth=Zero  SaturateOnIntegerOverflow=off  InputSameDT=off
  Unit Delay : UnitDelay  SampleTime=-1  HasFrameUpgradeWarning=on
  Out1 : Outport
  wires:
  Unit Delay/1 -> Sum1/1, Sum/1
  Gain/1 -> Sum/2
  Switch/1 -> Out1/1, Unit Delay/1
  Saturation/1 -> Sum1/2
  Sum/1 -> Saturation/1
  Constant1/1 -> Switch/3
  Open_Hz/1 -> Gain/1
  Sum1/1 -> Switch/1
  Reset/1 -> Switch/2

== system Senorless/FOC_PointModel/加速强拖/加速积分角度 ==
  Acc : Inport
  Data Type Conversion : DataTypeConversion  Commented=on  OutDataTypeStr=int16  SaturateOnIntegerOverflow=off
  Data Type Conversion1 : DataTypeConversion  Commented=on  OutDataTypeStr=int16  SaturateOnIntegerOverflow=off
  Data Type Conversion2 : DataTypeConversion  OutDataTypeStr=uint16  SaturateOnIntegerOverflow=off
  Data Type Conversion3 : DataTypeConversion  OutDataTypeStr=int32  SaturateOnIntegerOverflow=off
  Freq1 : InportShadow
  Gain6 : Gain  Commented=on  Gain=65535  OutDataTypeStr=int32  RndMeth=Zero
  Scope1 : Scope  Commented=on
  Scope2 : Scope  Commented=on
  Shift Arithmetic : ArithShift  BitShiftNumber=-16
  初始值1 : Constant  Commented=on  Value=0  OutDataTypeStr=int32
  初始值3 : Constant  Commented=on  Value=0  OutDataTypeStr=int32
  积分器 : Subsystem  Commented=on
  积分器2 : Subsystem  Commented=on
  积分器3 : Subsystem
      settings: MinAlgLoopOccurrences=on
  积分器4 : Subsystem
      settings: MinAlgLoopOccurrences=on
  积分增益 : Constant  Commented=on  Value=32767  OutDataTypeStr=int32
  积分增益1 : Constant  Commented=on  Value=32767  OutDataTypeStr=int32
  这是积分增益缩小 : ArithShift  Commented=on  BitShiftNumber=15
  这是积分增益缩小1 : ArithShift  Commented=on  BitShiftNumber=15
  Theta : Outport
  wires:
  Data Type Conversion1/1 -> Gain6/1
  Gain6/1 -> 积分器/2(input)
  积分增益/1 -> 积分器/1(K_p)
  初始值1/1 -> 积分器2/3(Xo)
  积分增益1/1 -> 积分器2/1(K_p)
  这是积分增益缩小1/1 -> Data Type Conversion/1
  积分器2/1(output) -> Scope1/1, 这是积分增益缩小/1
  积分器/1(output) -> Scope2/1, 积分器2/2(input)
  这是积分增益缩小/1 -> 这是积分增益缩小1/1
  Shift Arithmetic/1 -> 积分器3/1(input)
  Acc/1 -> Data Type Conversion3/1
  Freq1/1 -> Data Type Conversion1/1
  初始值3/1 -> 积分器/3(Xo)
  Data Type Conversion2/1 -> Theta/1
  积分器3/1(output) -> 积分器4/1(input)
  积分器4/1(output) -> Data Type Conversion2/1
  Data Type Conversion3/1 -> Shift Arithmetic/1
